simulink model "HDLOfdmDemod"  (R2024a)
settings: Solver=FixedStepDiscrete  StartTime=0.0  StopTime=stopTime  RelTol=1e-3
undefined symbols (not defined in the file): CONST, dataSymbols
libraries: dspsrcs4 x2, HDL_ieee_8021513 x2, hdlsllib x1, whdlutilities x1
settings Model: DataTypeOverride=Off  SimulationMode=accelerator  Creator=cotti  LastModifiedBy=cotti
settings OptimizationCC: BlockReduction=off  ConditionallyExecuteInputs=off  DefaultParameterBehavior=Inlined  InheritOutputTypeSmallerThanSingle=on
settings DebuggingCC: AlgebraicLoopMsg=error  ArtificialAlgebraicLoopMsg=error  SingleTaskRateTransMsg=error  UnconnectedInputMsg=warning  UnconnectedOutputMsg=warning  UnconnectedLineMsg=warning
settings HardwareCC: ProdBitPerPointer=32  ProdBitPerSizeT=32  ProdBitPerPtrDiffT=32  ProdLargestAtomicFloat=None  ProdIntDivRoundTo=Undefined  ProdEndianess=Unspecified  ProdWordSize=32  ProdHWDeviceType=ASIC/FPGA->ASIC/FPGA  TargetBitPerLong=64  TargetBitPerPointer=64  TargetBitPerSizeT=64  TargetBitPerPtrDiffT=64  TargetLongLongMode=on  TargetIntDivRoundTo=Zero  TargetEndianess=LittleEndian  TargetWordSize=64  TargetHWDeviceType=Custom Processor->MATLAB Host Computer  ProdEqTarget=off

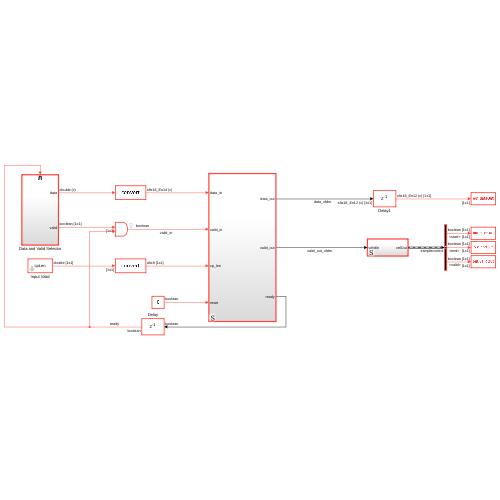
[thumbnail: Simulink's stored preview of the top-level diagram]
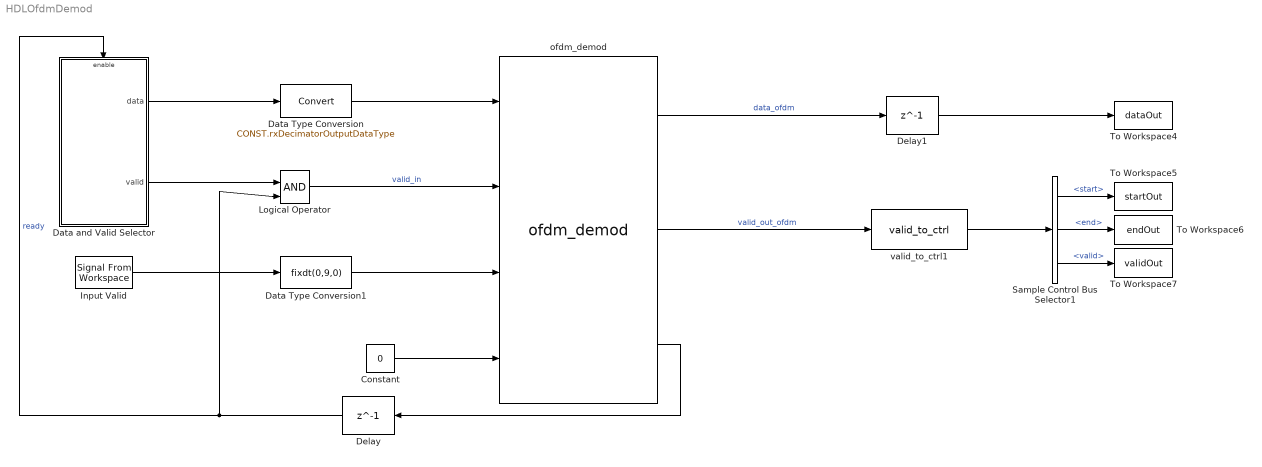
== system HDLOfdmDemod ==
  Constant : Constant  Value=0  OutDataTypeStr=boolean  SampleTime=1/CONST.fPHY
  Data Type Conversion : DataTypeConversion  OutDataTypeStr=CONST.rxDecimatorOutputDataType  SaturateOnIntegerOverflow=off  RndMeth=Floor
  Data Type Conversion1 : DataTypeConversion  OutDataTypeStr=fixdt(0,9,0)  SaturateOnIntegerOverflow=off  RndMeth=Floor
  Data and Valid Selector : Subsystem  TreatAsAtomicUnit=on
  Delay : Delay  DelayLength=1  InitialCondition=0  UseCircularBuffer=on
  Delay1 : Delay  DelayLength=1  InitialCondition=0  UseCircularBuffer=on
  Input Valid : dspsrcs4/Signal From Workspace  X=cpLen  Ts=1/CONST.fPHY  nsamps=1  OutputAfterFinalValue=Holding final value  ignoreOrWarnInputAndFrameLengths=off  OutputFrames=off
  Logical Operator : Logic  IconShape=distinctive  AllPortsSameDT=off  OutDataTypeStr=boolean
  Sample Control Bus Selector1 : whdlutilities/Sample Control Bus Selector  OutputSignals=start,end,valid
  To Workspace4 : ToWorkspace  VariableName=dataOut  SampleTime=1/CONST.fPHY
      settings: Save2DSignal=2-D array (concatenate along first dimension)
  To Workspace5 : ToWorkspace  VariableName=startOut  SampleTime=1/CONST.fPHY
      settings: Save2DSignal=2-D array (concatenate along first dimension)
  To Workspace6 : ToWorkspace  VariableName=endOut  SampleTime=1/CONST.fPHY
      settings: Save2DSignal=2-D array (concatenate along first dimension)
  To Workspace7 : ToWorkspace  VariableName=validOut  SampleTime=1/CONST.fPHY
      settings: Save2DSignal=2-D array (concatenate along first dimension)
  ofdm_demod : HDL_ieee_8021513/ofdm_demod  SystemSampleTime=-1  VariantActivationTime=update diagram  AllowFlexibleInterface=on  Latency=0  AutoFrameSizeCalculation=off
      settings: SourceProductName=HDL IEEE 8021513
  valid_to_ctrl1 : HDL_ieee_8021513/valid_to_ctrl  SystemSampleTime=-1  VariantActivationTime=update diagram  AllowFlexibleInterface=on  Latency=0  AutoFrameSizeCalculation=off
      settings: SourceProductName=HDL IEEE 8021513
  wires:
  Delay1/1 -> To Workspace4/1
  ofdm_demod/2 -> valid_to_ctrl1/1  "valid_out_ofdm"
  Sample Control Bus Selector1/1 -> To Workspace5/1  "<start>"
  ofdm_demod/1 -> Delay1/1  "data_ofdm"
  Sample Control Bus Selector1/3 -> To Workspace7/1  "<valid>"
  Sample Control Bus Selector1/2 -> To Workspace6/1  "<end>"
  valid_to_ctrl1/1 -> Sample Control Bus Selector1/1
  ofdm_demod/3 -> Delay/1
  Data and Valid Selector/1(data) -> Data Type Conversion/1
  Data and Valid Selector/2(valid) -> Logical Operator/1
  Delay/1 -> Logical Operator/2, Data and Valid Selector/Enable  "ready"
  Logical Operator/1 -> ofdm_demod/2  "valid_in"
  Input Valid/1 -> Data Type Conversion1/1
  Data Type Conversion/1 -> ofdm_demod/1
  Constant/1 -> ofdm_demod/4
  Data Type Conversion1/1 -> ofdm_demod/3

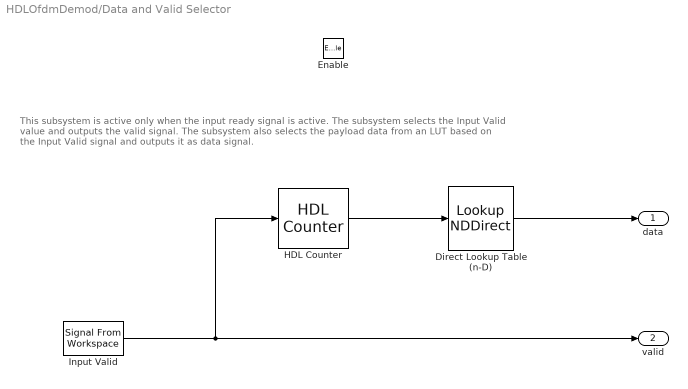
== system HDLOfdmDemod/Data and Valid Selector ==
  note: This subsystem is active only when the input ready signal is active. The subsystem selects the Input Valid value and outputs the valid signal.
      | The subsystem also selects the payload data from an LUT based on the Input Valid signal and outputs it as data signal.
  Enable : EnablePort
  Direct Lookup Table (n-D) : LookupNDDirect  NumberOfTableDimensions=1  Table=dataSymbols  DiagnosticForOutOfRangeInput=Error  TableDataTypeStr=double
  HDL Counter : hdlsllib/Sources/HDL Counter  CountType=Count limited  CountInit=0  CountStep=1  CountMax=length(dataSymbols) -1  CountFromType=Initial value  CountFrom=0  CountResetPort=off  CountLoadPort=off  CountEnbPort=on  CountDirPort=off  CountHitOutputPort=off  CountDataType=Unsigned  CountWordLen=nextpow2(length(dataSymbols))  CountFracLen=0  CountSampTime=1
  Input Valid : dspsrcs4/Signal From Workspace  X=validIn  Ts=1/CONST.fPHY  nsamps=1  OutputAfterFinalValue=Setting to zero  ignoreOrWarnInputAndFrameLengths=off  OutputFrames=off
  data : Outport  InitialOutput=0  VectorParamsAs1DForOutWhenUnconnected=off
  valid : Outport  Port=2  InitialOutput=0  VectorParamsAs1DForOutWhenUnconnected=off
  wires:
  HDL Counter/1 -> Direct Lookup Table (n-D)/1
  Input Valid/1 -> HDL Counter/1, valid/1
  Direct Lookup Table (n-D)/1 -> data/1
